simulink model "r"  (Simulink 7.5)
settings: Solver=ode1  StartTime=0.0  StopTime=inf  FixedStep=0.02  RelTol=1e-3
undefined symbols (not defined in the file): Standard_Devices, UDP_Protocol
libraries: simulink x19, rtwinlib x2
settings Model: Creator=dagothar  LastModifiedBy=dagothar  SimulationMode=external  ExtModeBatchMode=on
settings DebuggingCC: MultiTaskRateTransMsg=warning
settings HardwareCC: ProdIntDivRoundTo=Zero  ProdEndianess=LittleEndian  ProdHWDeviceType=Generic->32-bit x86 compatible
settings RTWCC: SystemTargetFile=rtwin.tlc  TemplateMakefile=rtwin.tmf  Description=Real-Time Windows Target  ProcessScript=rtwin_make_rtw_hook  RTWCompilerOptimization=On
settings CodeAppCC: MaxIdLength=95
settings RTWinTargetCC: TargetLibSuffix=_rtwin.lib  TargetPreCompLibLocation=d:\Program Files\MATLAB\R2010a\toolbox\rtw\targets\rtwin\lib  TargetFunctionLibrary=ANSI_C  ERTCodeCoverageTool=None  PortableWordSizes=off

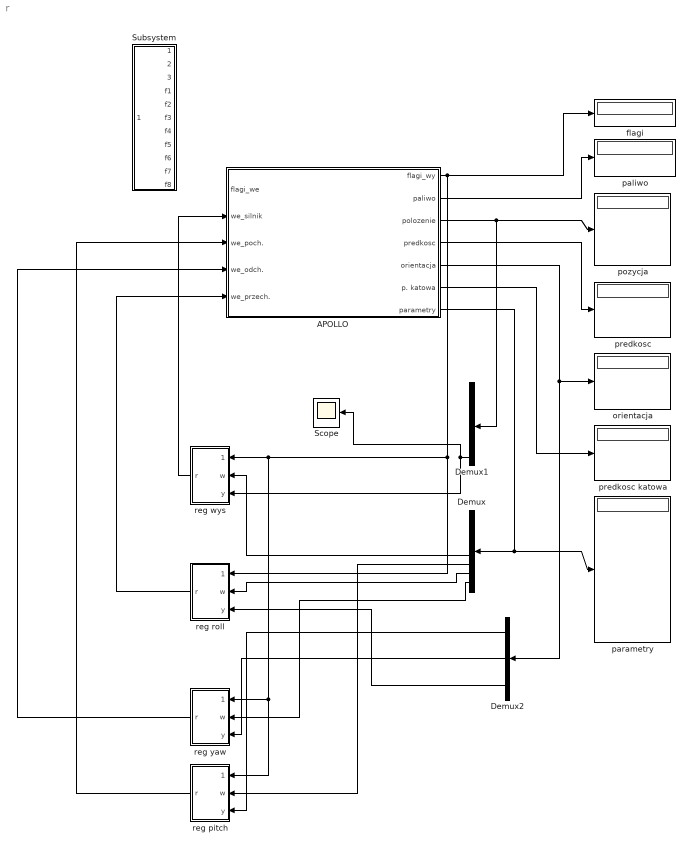
== system r ==
  APOLLO : Subsystem  mask(Interfejs programu APOLLO){dt_recv=0.02, dt_send=0.02}
      mask prompts: dt_recv "Co ile odbierac dane?"; dt_send "Co ile wysylac dane?"
      mask help:
      | Nawiazuje komunikacje poprzez protokol UDP z symulatorem APOLLO uruchomionym na lokalnym komputerze.
      | Umozliwia sterowanie stanem ladownika, silnikiem glownym i silnikami systemu kontroli rotacji.
      | Zwraca aktualny stan ladownika.
      mask Display:
      | %pokaz obrazek
      | image(imread('simulink_data/apollo_icon.bmp'), 'center')
      | 
      | %oznaczenia portow
      | port_label('input', 1, 'we. flagi')
      | port_label('input', 2, 'we. silnik')
      | port_label('input', 3, 'we. poch.')
      | port_label('input', 4, 'we. odch.')
      | port_label('input', 5, 'we. przech.')
      | port_label('output', 1, 'wy. flagi')
      | port_label('output', 2, 'paliwo')
      | port_label('output', 3, 'pozycja')
      | port_label('output', 4, 'predkosc')
      | port_label('output', 5, 'orientacja')
      | port_label('output', 6, 'p. katowa')
      | port_label('output', 7, 'parametry')
  Demux : Demux  Outputs=8
  Demux1 : Demux
  Demux2 : Demux  Outputs=3
  Scope : Scope
      settings: YMin=0  YMax=13
  Subsystem : Subsystem
  flagi : Display
  orientacja : Display
  paliwo : Display
  parametry : Display
  pozycja : Display
  predkosc : Display
  predkosc katowa : Display
  reg pitch : Subsystem  mask{enable_mask=bin2dec('1000000000'), kp=0.012, ki=0.000001, kd=0.07}
      mask prompts: enable_mask "Maska bitu wlaczenia:"
  reg roll : Subsystem  mask{enable_mask=bin2dec('10000000000'), kp=0.012, ki=0.000001, kd=0.07}
      mask prompts: enable_mask "Maska bitu wlaczenia:"
  reg wys : Subsystem  mask{enable_mask=bin2dec('100000000'), kp=0.15, ki=0.01, kd=0.5}
      mask prompts: enable_mask "Maska bitu wlaczenia:"
  reg yaw : Subsystem  mask{enable_mask=bin2dec('100000000000'), kp=0.012, ki=0.000001, kd=0.07}
      mask prompts: enable_mask "Maska bitu wlaczenia:"
  wires:
  APOLLO/2(paliwo) -> paliwo/1
  APOLLO/3(polozenie) -> pozycja/1, Demux1/1
  APOLLO/5(orientacja) -> orientacja/1, Demux2/1
  APOLLO/6(p. katowa) -> predkosc katowa/1
  APOLLO/4(predkosc) -> predkosc/1
  APOLLO/7(parametry) -> parametry/1, Demux/1
  APOLLO/1(flagi_wy) -> flagi/1, reg roll/1(enable), reg wys/1(enable), reg yaw/1(enable), reg pitch/1(enable)
  reg wys/1(r) -> APOLLO/2(we_silnik)
  Demux/5 -> reg wys/2(w)
  reg roll/1(r) -> APOLLO/5(we_przech.)
  Demux2/3 -> reg roll/3(y)
  reg yaw/1(r) -> APOLLO/4(we_odch.)
  Demux2/2 -> reg yaw/3(y)
  Demux1/4 -> Scope/1, reg wys/3(y)
  Demux/7 -> reg roll/2(w)
  Demux/8 -> reg yaw/2(w)
  reg pitch/1(r) -> APOLLO/3(we_poch.)
  Demux/6 -> reg pitch/2(w)
  Demux2/1 -> reg pitch/3(y)

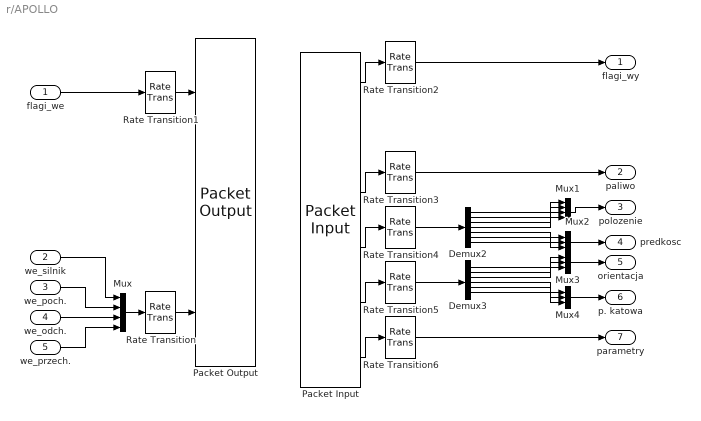
== system r/APOLLO ==
  flagi_we : Inport  OutDataType=fixdt(1, 16)  OutScaling=2^0
  we_silnik : Inport  Port=2  OutDataType=fixdt(1, 16)  OutScaling=2^0
  we_poch. : Inport  Port=3  OutDataType=fixdt(1, 16)  OutScaling=2^0
  we_odch. : Inport  Port=4  OutDataType=fixdt(1, 16)  OutScaling=2^0
  we_przech. : Inport  Port=5  OutDataType=fixdt(1, 16)  OutScaling=2^0
  Demux2 : Demux  Outputs=7
  Demux3 : Demux  Outputs=6
  Mux : Mux
  Mux1 : Mux
  Mux2 : Mux  Inputs=3
  Mux3 : Mux  Inputs=3
  Mux4 : Mux  Inputs=3
  Packet Input : rtwinlib/Packet Input  SampleTime=dt_recv  DrvName=Standard_Devices/UDP_Protocol  DrvAddress=12001  DrvOptions=[2130706433 12000]  PacketSize=192  DataTypes="{'int32', 'int32',  '2*double', '7*double', '6*double', '8*double'}"  ShowReady=off  ShowError=off  PacketID=1  ShowTimestamp=off
      settings: AttributesFormatString=Standard Devices\nUDP Protocol [2EE1h]
  Packet Output : rtwinlib/Packet Output  SampleTime=dt_send  DrvName=Standard_Devices/UDP_Protocol  DrvAddress=12002  DrvOptions=[2130706433 12003]  PacketSize=40  DataTypes={'int32', 'int32', '4*double'}  ShowReady=off  ShowError=off  PacketID=1  InitialValue=[]  FinalValue=[]
      settings: AttributesFormatString=Standard Devices\nUDP Protocol [2EE2h]
  Rate Transition{,1..6} (7 alike) : RateTransition
  flagi_wy : Outport  OutDataType=fixdt(1, 16)  OutScaling=2^0
  paliwo : Outport  Port=2  OutDataType=fixdt(1, 16)  OutScaling=2^0
  polozenie : Outport  Port=3  OutDataType=fixdt(1, 16)  OutScaling=2^0
  predkosc : Outport  Port=4  OutDataType=fixdt(1, 16)  OutScaling=2^0
  orientacja : Outport  Port=5  OutDataType=fixdt(1, 16)  OutScaling=2^0
  p. katowa : Outport  Port=6  OutDataType=fixdt(1, 16)  OutScaling=2^0
  parametry : Outport  Port=7  OutDataType=fixdt(1, 16)  OutScaling=2^0
  wires:
  Packet Input/4 -> Rate Transition4/1
  Packet Input/5 -> Rate Transition5/1
  Packet Input/6 -> Rate Transition6/1
  Packet Input/3 -> Rate Transition3/1
  Packet Input/1 -> Rate Transition2/1
  Demux2/1 -> Mux1/1
  Demux2/2 -> Mux1/2
  Demux2/3 -> Mux1/3
  Mux1/1 -> polozenie/1
  Mux2/1 -> predkosc/1
  Demux3/1 -> Mux3/1
  Demux3/2 -> Mux3/2
  Demux3/3 -> Mux3/3
  Mux3/1 -> orientacja/1
  Demux3/4 -> Mux4/1
  Demux3/5 -> Mux4/2
  Demux3/6 -> Mux4/3
  Mux4/1 -> p. katowa/1
  Mux/1 -> Rate Transition/1
  flagi_we/1 -> Rate Transition1/1
  we_odch./1 -> Mux/3
  we_poch./1 -> Mux/2
  we_silnik/1 -> Mux/1
  we_przech./1 -> Mux/4
  Rate Transition/1 -> Packet Output/3
  Rate Transition1/1 -> Packet Output/1
  Rate Transition2/1 -> flagi_wy/1
  Rate Transition3/1 -> paliwo/1
  Rate Transition4/1 -> Demux2/1
  Rate Transition5/1 -> Demux3/1
  Rate Transition6/1 -> parametry/1
  Demux2/5 -> Mux2/1
  Demux2/4 -> Mux1/4
  Demux2/6 -> Mux2/2
  Demux2/7 -> Mux2/3

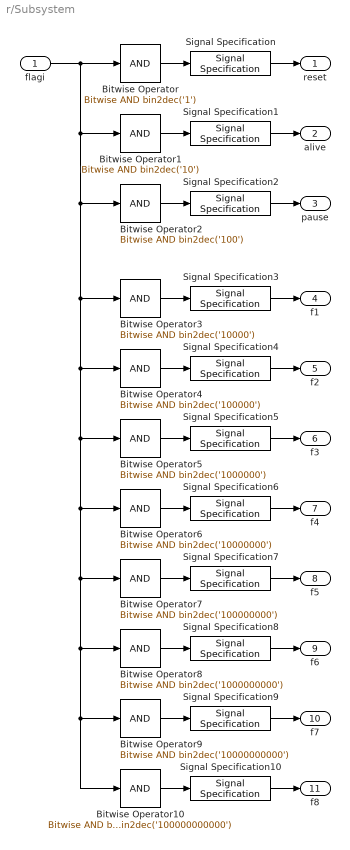
== system r/Subsystem ==
  flagi : Inport  OutDataType=fixdt(1, 16)  OutScaling=2^0
  Bitwise Operator : simulink/Logic and Bit Operations/Bitwise Operator  logicop=AND  UseBitMask=on  BitMask=bin2dec('1')  BitMaskRealWorld=Stored Integer
  Bitwise Operator1 : simulink/Logic and Bit Operations/Bitwise Operator  logicop=AND  UseBitMask=on  BitMask=bin2dec('10')  BitMaskRealWorld=Stored Integer
  Bitwise Operator10 : simulink/Logic and Bit Operations/Bitwise Operator  logicop=AND  UseBitMask=on  BitMask=bin2dec('100000000000')  BitMaskRealWorld=Stored Integer
  Bitwise Operator2 : simulink/Logic and Bit Operations/Bitwise Operator  logicop=AND  UseBitMask=on  BitMask=bin2dec('100')  BitMaskRealWorld=Stored Integer
  Bitwise Operator3 : simulink/Logic and Bit Operations/Bitwise Operator  logicop=AND  UseBitMask=on  BitMask=bin2dec('10000')  BitMaskRealWorld=Stored Integer
  Bitwise Operator4 : simulink/Logic and Bit Operations/Bitwise Operator  logicop=AND  UseBitMask=on  BitMask=bin2dec('100000')  BitMaskRealWorld=Stored Integer
  Bitwise Operator5 : simulink/Logic and Bit Operations/Bitwise Operator  logicop=AND  UseBitMask=on  BitMask=bin2dec('1000000')  BitMaskRealWorld=Stored Integer
  Bitwise Operator6 : simulink/Logic and Bit Operations/Bitwise Operator  logicop=AND  UseBitMask=on  BitMask=bin2dec('10000000')  BitMaskRealWorld=Stored Integer
  Bitwise Operator7 : simulink/Logic and Bit Operations/Bitwise Operator  logicop=AND  UseBitMask=on  BitMask=bin2dec('100000000')  BitMaskRealWorld=Stored Integer
  Bitwise Operator8 : simulink/Logic and Bit Operations/Bitwise Operator  logicop=AND  UseBitMask=on  BitMask=bin2dec('1000000000')  BitMaskRealWorld=Stored Integer
  Bitwise Operator9 : simulink/Logic and Bit Operations/Bitwise Operator  logicop=AND  UseBitMask=on  BitMask=bin2dec('10000000000')  BitMaskRealWorld=Stored Integer
  Signal Specification{,1..10} (11 alike) : SignalSpecification  DataType=boolean  OutDataType=fixdt(1, 16)  OutScaling=2^0  OutDataTypeStr=boolean
  reset : Outport  OutDataType=fixdt(1, 16)  OutScaling=2^0
  alive : Outport  Port=2  OutDataType=fixdt(1, 16)  OutScaling=2^0
  pause : Outport  Port=3  OutDataType=fixdt(1, 16)  OutScaling=2^0
  f1 : Outport  Port=4  OutDataType=fixdt(1, 16)  OutScaling=2^0
  f2 : Outport  Port=5  OutDataType=fixdt(1, 16)  OutScaling=2^0
  f3 : Outport  Port=6  OutDataType=fixdt(1, 16)  OutScaling=2^0
  f4 : Outport  Port=7  OutDataType=fixdt(1, 16)  OutScaling=2^0
  f5 : Outport  Port=8  OutDataType=fixdt(1, 16)  OutScaling=2^0
  f6 : Outport  Port=9  OutDataType=fixdt(1, 16)  OutScaling=2^0
  f7 : Outport  Port=10  OutDataType=fixdt(1, 16)  OutScaling=2^0
  f8 : Outport  Port=11  OutDataType=fixdt(1, 16)  OutScaling=2^0
  wires:
  Bitwise Operator/1 -> Signal Specification/1
  Signal Specification/1 -> reset/1
  Bitwise Operator1/1 -> Signal Specification1/1
  Signal Specification1/1 -> alive/1
  Bitwise Operator2/1 -> Signal Specification2/1
  Signal Specification2/1 -> pause/1
  Bitwise Operator3/1 -> Signal Specification3/1
  Signal Specification3/1 -> f1/1
  Bitwise Operator4/1 -> Signal Specification4/1
  Signal Specification4/1 -> f2/1
  Bitwise Operator5/1 -> Signal Specification5/1
  Signal Specification5/1 -> f3/1
  Bitwise Operator6/1 -> Signal Specification6/1
  Signal Specification6/1 -> f4/1
  Bitwise Operator7/1 -> Signal Specification7/1
  Signal Specification7/1 -> f5/1
  Bitwise Operator8/1 -> Signal Specification8/1
  Signal Specification8/1 -> f6/1
  Bitwise Operator9/1 -> Signal Specification9/1
  Signal Specification9/1 -> f7/1
  Bitwise Operator10/1 -> Signal Specification10/1
  Signal Specification10/1 -> f8/1
  flagi/1 -> Bitwise Operator/1, Bitwise Operator1/1, Bitwise Operator2/1, Bitwise Operator3/1, Bitwise Operator4/1, Bitwise Operator5/1, Bitwise Operator6/1, Bitwise Operator7/1, Bitwise Operator8/1, Bitwise Operator9/1, Bitwise Operator10/1

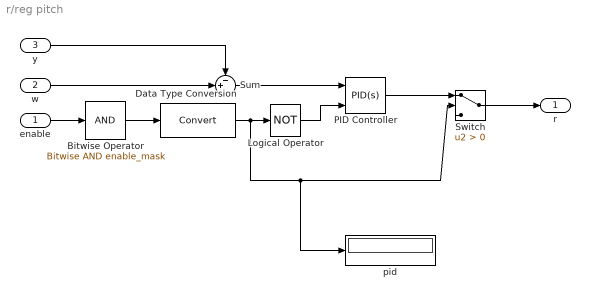
== system r/reg pitch ==
  enable : Inport  OutDataType=fixdt(1, 16)  OutScaling=2^0
  w : Inport  Port=2  OutDataType=fixdt(1, 16)  OutScaling=2^0
  y : Inport  Port=3  OutDataType=fixdt(1, 16)  OutScaling=2^0
  Bitwise Operator : simulink/Logic and Bit Operations/Bitwise Operator  logicop=AND  UseBitMask=on  BitMask=enable_mask  BitMaskRealWorld=Stored Integer
  Data Type Conversion : DataTypeConversion  OutDataType=fixdt(1, 16)  OutScaling=2^0
  Logical Operator : Logic  Operator=NOT  AllPortsSameDT=off  OutDataTypeMode=boolean  LogicDataType=fixdt(0, 8)  OutDataTypeStr=boolean
  PID Controller : simulink/Continuous/PID Controller  DialogController=pidpack.PIDConfig.pidDDGCreate  DialogControllerArgs=DataTag0  SystemSampleTime=-1  Controller=PID  TimeDomain=Continuous-time  SampleTime=1  IntegratorMethod=Forward Euler  FilterMethod=Forward Euler  Form=Parallel  P=kp  I=ki  D=kd  N=10  InitialConditionSource=internal  InitialConditionForIntegrator=0  InitialConditionForFilter=0  ExternalReset=level  LimitOutput=off  UpperSaturationLimit=inf  LowerSaturationLimit=-inf  LinearizeAsGain=off  AntiWindupMode=none  Kb=1  TrackingMode=off  Kt=1  PParamMin=[]  PParamMax=[]  IParamMin=[]  IParamMax=[]  DParamMin=[]  DParamMax=[]  NParamMin=[]  NParamMax=[]  KbParamMin=[]  KbParamMax=[]  KtParamMin=[]  KtParamMax=[]  POutMin=[]  POutMax=[]  IOutMin=[]  IOutMax=[]  DOutMin=[]  DOutMax=[]  NOutMin=[]  NOutMax=[]  KbOutMin=[]  KbOutMax=[]  KtOutMin=[]  KtOutMax=[]  IntegratorOutMin=[]  IntegratorOutMax=[]  FilterOutMin=[]  FilterOutMax=[]  SumOutMin=[]  SumOutMax=[]  SumI1OutMin=[]  SumI1OutMax=[]  SumI2OutMin=[]  SumI2OutMax=[]  SumI3OutMin=[]  SumI3OutMax=[]  SumDOutMin=[]  SumDOutMax=[]  SaturationOutMin=[]  SaturationOutMax=[]  IntegratorContinuousStateAttributes=''  IntegratorStateMustResolveToSignalObject=off  IntegratorRTWStateStorageClass=Auto  FilterContinuousStateAttributes=''  FilterStateMustResolveToSignalObject=off  FilterRTWStateStorageClass=Auto
  Sum : Sum  Inputs=-+|  OutDataType=fixdt(1, 16)  OutScaling=2^0
  Switch : Switch  Criteria=u2 > Threshold  OutDataType=fixdt(1, 16)  OutScaling=2^0
  pid : Display
  r : Outport  OutDataType=fixdt(1, 16)  OutScaling=2^0
  wires:
  Bitwise Operator/1 -> Data Type Conversion/1
  Sum/1 -> PID Controller/1
  Data Type Conversion/1 -> Logical Operator/1, Switch/2, pid/1
  w/1 -> Sum/2
  y/1 -> Sum/1
  enable/1 -> Bitwise Operator/1
  Logical Operator/1 -> PID Controller/2
  PID Controller/1 -> Switch/1
  Switch/1 -> r/1

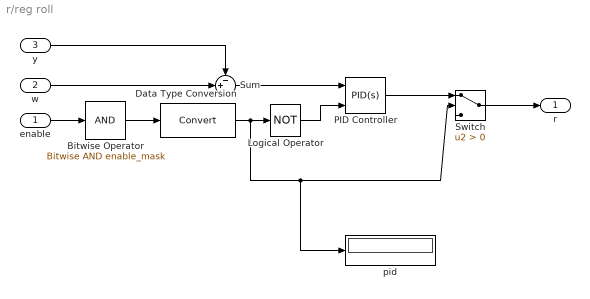
== system r/reg roll ==
  enable : Inport  OutDataType=fixdt(1, 16)  OutScaling=2^0
  w : Inport  Port=2  OutDataType=fixdt(1, 16)  OutScaling=2^0
  y : Inport  Port=3  OutDataType=fixdt(1, 16)  OutScaling=2^0
  Bitwise Operator : simulink/Logic and Bit Operations/Bitwise Operator  logicop=AND  UseBitMask=on  BitMask=enable_mask  BitMaskRealWorld=Stored Integer
  Data Type Conversion : DataTypeConversion  OutDataType=fixdt(1, 16)  OutScaling=2^0
  Logical Operator : Logic  Operator=NOT  AllPortsSameDT=off  OutDataTypeMode=boolean  LogicDataType=fixdt(0, 8)  OutDataTypeStr=boolean
  PID Controller : simulink/Continuous/PID Controller  DialogController=pidpack.PIDConfig.pidDDGCreate  DialogControllerArgs=DataTag1  SystemSampleTime=-1  Controller=PID  TimeDomain=Continuous-time  SampleTime=1  IntegratorMethod=Forward Euler  FilterMethod=Forward Euler  Form=Parallel  P=kp  I=ki  D=kd  N=10  InitialConditionSource=internal  InitialConditionForIntegrator=0  InitialConditionForFilter=0  ExternalReset=level  LimitOutput=off  UpperSaturationLimit=inf  LowerSaturationLimit=-inf  LinearizeAsGain=off  AntiWindupMode=none  Kb=1  TrackingMode=off  Kt=1  PParamMin=[]  PParamMax=[]  IParamMin=[]  IParamMax=[]  DParamMin=[]  DParamMax=[]  NParamMin=[]  NParamMax=[]  KbParamMin=[]  KbParamMax=[]  KtParamMin=[]  KtParamMax=[]  POutMin=[]  POutMax=[]  IOutMin=[]  IOutMax=[]  DOutMin=[]  DOutMax=[]  NOutMin=[]  NOutMax=[]  KbOutMin=[]  KbOutMax=[]  KtOutMin=[]  KtOutMax=[]  IntegratorOutMin=[]  IntegratorOutMax=[]  FilterOutMin=[]  FilterOutMax=[]  SumOutMin=[]  SumOutMax=[]  SumI1OutMin=[]  SumI1OutMax=[]  SumI2OutMin=[]  SumI2OutMax=[]  SumI3OutMin=[]  SumI3OutMax=[]  SumDOutMin=[]  SumDOutMax=[]  SaturationOutMin=[]  SaturationOutMax=[]  IntegratorContinuousStateAttributes=''  IntegratorStateMustResolveToSignalObject=off  IntegratorRTWStateStorageClass=Auto  FilterContinuousStateAttributes=''  FilterStateMustResolveToSignalObject=off  FilterRTWStateStorageClass=Auto
  Sum : Sum  Inputs=-+|  OutDataType=fixdt(1, 16)  OutScaling=2^0
  Switch : Switch  Criteria=u2 > Threshold  OutDataType=fixdt(1, 16)  OutScaling=2^0
  pid : Display
  r : Outport  OutDataType=fixdt(1, 16)  OutScaling=2^0
  wires:
  Bitwise Operator/1 -> Data Type Conversion/1
  Sum/1 -> PID Controller/1
  Data Type Conversion/1 -> Logical Operator/1, Switch/2, pid/1
  w/1 -> Sum/2
  y/1 -> Sum/1
  enable/1 -> Bitwise Operator/1
  Logical Operator/1 -> PID Controller/2
  PID Controller/1 -> Switch/1
  Switch/1 -> r/1

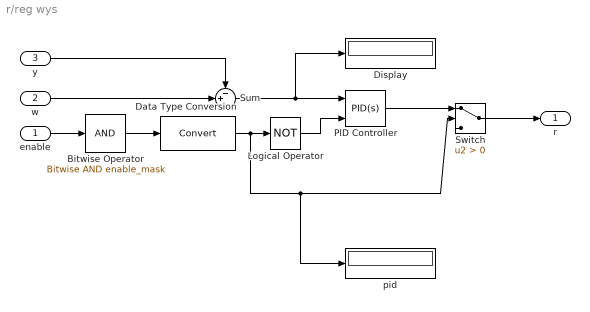
== system r/reg wys ==
  enable : Inport  OutDataType=fixdt(1, 16)  OutScaling=2^0
  w : Inport  Port=2  OutDataType=fixdt(1, 16)  OutScaling=2^0
  y : Inport  Port=3  OutDataType=fixdt(1, 16)  OutScaling=2^0
  Bitwise Operator : simulink/Logic and Bit Operations/Bitwise Operator  logicop=AND  UseBitMask=on  BitMask=enable_mask  BitMaskRealWorld=Stored Integer
  Data Type Conversion : DataTypeConversion  OutDataType=fixdt(1, 16)  OutScaling=2^0
  Display : Display
  Logical Operator : Logic  Operator=NOT  AllPortsSameDT=off  OutDataTypeMode=boolean  LogicDataType=fixdt(0, 8)  OutDataTypeStr=boolean
  PID Controller : simulink/Continuous/PID Controller  DialogController=pidpack.PIDConfig.pidDDGCreate  DialogControllerArgs=DataTag2  SystemSampleTime=-1  Controller=PID  TimeDomain=Continuous-time  SampleTime=1  IntegratorMethod=Forward Euler  FilterMethod=Forward Euler  Form=Parallel  P=kp  I=ki  D=kd  N=10  InitialConditionSource=internal  InitialConditionForIntegrator=0  InitialConditionForFilter=0  ExternalReset=level  LimitOutput=off  UpperSaturationLimit=inf  LowerSaturationLimit=-inf  LinearizeAsGain=off  AntiWindupMode=none  Kb=1  TrackingMode=off  Kt=1  PParamMin=[]  PParamMax=[]  IParamMin=[]  IParamMax=[]  DParamMin=[]  DParamMax=[]  NParamMin=[]  NParamMax=[]  KbParamMin=[]  KbParamMax=[]  KtParamMin=[]  KtParamMax=[]  POutMin=[]  POutMax=[]  IOutMin=[]  IOutMax=[]  DOutMin=[]  DOutMax=[]  NOutMin=[]  NOutMax=[]  KbOutMin=[]  KbOutMax=[]  KtOutMin=[]  KtOutMax=[]  IntegratorOutMin=[]  IntegratorOutMax=[]  FilterOutMin=[]  FilterOutMax=[]  SumOutMin=[]  SumOutMax=[]  SumI1OutMin=[]  SumI1OutMax=[]  SumI2OutMin=[]  SumI2OutMax=[]  SumI3OutMin=[]  SumI3OutMax=[]  SumDOutMin=[]  SumDOutMax=[]  SaturationOutMin=[]  SaturationOutMax=[]  IntegratorContinuousStateAttributes=''  IntegratorStateMustResolveToSignalObject=off  IntegratorRTWStateStorageClass=Auto  FilterContinuousStateAttributes=''  FilterStateMustResolveToSignalObject=off  FilterRTWStateStorageClass=Auto
  Sum : Sum  Inputs=-+|  OutDataType=fixdt(1, 16)  OutScaling=2^0
  Switch : Switch  Criteria=u2 > Threshold  OutDataType=fixdt(1, 16)  OutScaling=2^0
  pid : Display
  r : Outport  OutDataType=fixdt(1, 16)  OutScaling=2^0
  wires:
  Bitwise Operator/1 -> Data Type Conversion/1
  Sum/1 -> PID Controller/1, Display/1
  Data Type Conversion/1 -> Logical Operator/1, Switch/2, pid/1
  w/1 -> Sum/2
  y/1 -> Sum/1
  enable/1 -> Bitwise Operator/1
  Logical Operator/1 -> PID Controller/2
  PID Controller/1 -> Switch/1
  Switch/1 -> r/1

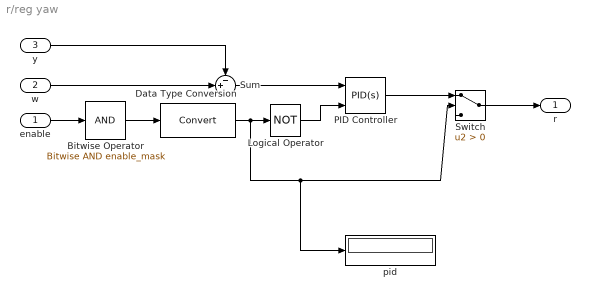
== system r/reg yaw ==
  enable : Inport  OutDataType=fixdt(1, 16)  OutScaling=2^0
  w : Inport  Port=2  OutDataType=fixdt(1, 16)  OutScaling=2^0
  y : Inport  Port=3  OutDataType=fixdt(1, 16)  OutScaling=2^0
  Bitwise Operator : simulink/Logic and Bit Operations/Bitwise Operator  logicop=AND  UseBitMask=on  BitMask=enable_mask  BitMaskRealWorld=Stored Integer
  Data Type Conversion : DataTypeConversion  OutDataType=fixdt(1, 16)  OutScaling=2^0
  Logical Operator : Logic  Operator=NOT  AllPortsSameDT=off  OutDataTypeMode=boolean  LogicDataType=fixdt(0, 8)  OutDataTypeStr=boolean
  PID Controller : simulink/Continuous/PID Controller  DialogController=pidpack.PIDConfig.pidDDGCreate  DialogControllerArgs=DataTag3  SystemSampleTime=-1  Controller=PID  TimeDomain=Continuous-time  SampleTime=1  IntegratorMethod=Forward Euler  FilterMethod=Forward Euler  Form=Parallel  P=kp  I=ki  D=kd  N=10  InitialConditionSource=internal  InitialConditionForIntegrator=0  InitialConditionForFilter=0  ExternalReset=level  LimitOutput=off  UpperSaturationLimit=inf  LowerSaturationLimit=-inf  LinearizeAsGain=off  AntiWindupMode=none  Kb=1  TrackingMode=off  Kt=1  PParamMin=[]  PParamMax=[]  IParamMin=[]  IParamMax=[]  DParamMin=[]  DParamMax=[]  NParamMin=[]  NParamMax=[]  KbParamMin=[]  KbParamMax=[]  KtParamMin=[]  KtParamMax=[]  POutMin=[]  POutMax=[]  IOutMin=[]  IOutMax=[]  DOutMin=[]  DOutMax=[]  NOutMin=[]  NOutMax=[]  KbOutMin=[]  KbOutMax=[]  KtOutMin=[]  KtOutMax=[]  IntegratorOutMin=[]  IntegratorOutMax=[]  FilterOutMin=[]  FilterOutMax=[]  SumOutMin=[]  SumOutMax=[]  SumI1OutMin=[]  SumI1OutMax=[]  SumI2OutMin=[]  SumI2OutMax=[]  SumI3OutMin=[]  SumI3OutMax=[]  SumDOutMin=[]  SumDOutMax=[]  SaturationOutMin=[]  SaturationOutMax=[]  IntegratorContinuousStateAttributes=''  IntegratorStateMustResolveToSignalObject=off  IntegratorRTWStateStorageClass=Auto  FilterContinuousStateAttributes=''  FilterStateMustResolveToSignalObject=off  FilterRTWStateStorageClass=Auto
  Sum : Sum  Inputs=-+|  OutDataType=fixdt(1, 16)  OutScaling=2^0
  Switch : Switch  Criteria=u2 > Threshold  OutDataType=fixdt(1, 16)  OutScaling=2^0
  pid : Display
  r : Outport  OutDataType=fixdt(1, 16)  OutScaling=2^0
  wires:
  Bitwise Operator/1 -> Data Type Conversion/1
  Sum/1 -> PID Controller/1
  Data Type Conversion/1 -> Logical Operator/1, Switch/2, pid/1
  w/1 -> Sum/2
  y/1 -> Sum/1
  enable/1 -> Bitwise Operator/1
  Logical Operator/1 -> PID Controller/2
  PID Controller/1 -> Switch/1
  Switch/1 -> r/1
